simulink model "mp"  (R2017b)
settings: Solver=FixedStepAuto  StartTime=0.0  StopTime=0  FixedStep=stepSize  RelTol=1e-3
InitFcn:
  | mp_init
values from neighbouring files (symbols this model uses):
  carrierFreq = 5e6    (= 5000000)    [mp_init.m]
  dataRate = 1e6    (= 1000000)    [mp_init.m]
  detection_threshold = 150 + 2^11    (= 2198)    [mp_init.m]
  memSize = 1024    [mp_init.m]
  pilot_size = 2    [mp_init.m]
  sampleRate = clockRate    (= 40000000)    [mp_init.m]
  stepSize = 1/sampleRate    (= 2.5e-08)    [mp_init.m]
  wordLength = 12    [mp_init.m]
undefined symbols (not defined in the file or in its folder): AdvDSPBChannelOutDisplay, AdvDSPBDMemDisplay, dpoly, dspba_ChannelInVis, dspba_ChannelOutVis, dspba_internal_get_channel_ports, evalAionMaskParam, latency, UseDontCare, value
libraries: DSPBAPrim x75, DSPBABase x13, DSPBAControl x10, DSPBAFilters x3
(part 2 of 2)

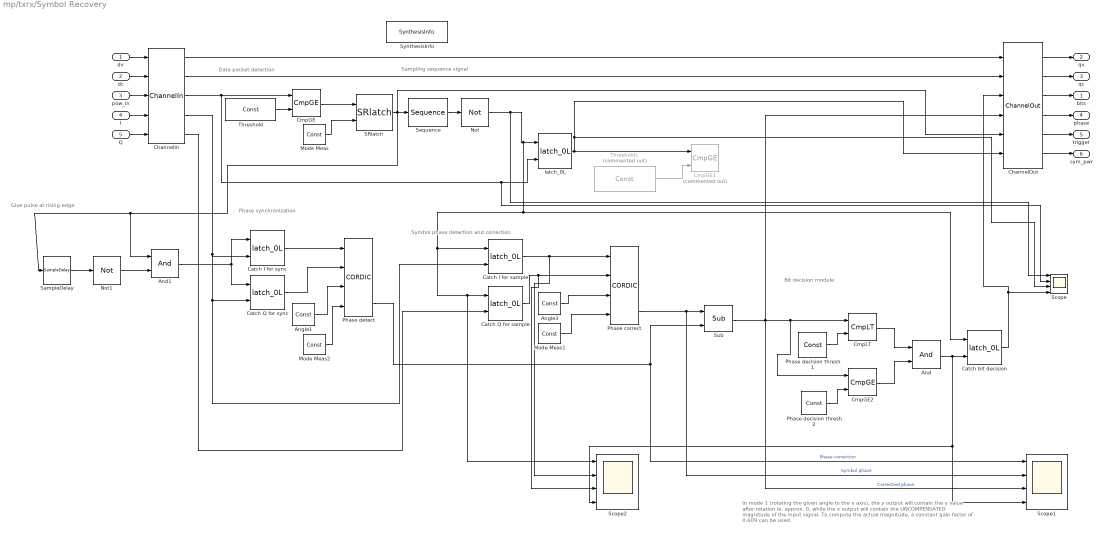
== system mp/txrx/Symbol Recovery ==
  note: Give pulse at rising edge
  note: Bit decision module
  note: Sampling sequence signal
  note: Data packet detection
  note: Symbol phase detection and correction
  note: Phase synchronization
  note: In mode 1 (rotating the given angle to the x axis),
      | the y output will contain the y value after rotation ie. approx. 0,
      | while the x output will contain the UNCOMPENSATED magnitude of the input signal.
      |
      | To compute the actual magnitude, a constant gain factor of 0.609 can be used.
  dv : Inport
  dc : Inport  Port=2
  pow_in : Inport  Port=3
  I : Inport  Port=4
  Q : Inport  Port=5
  And : DSPBAPrim/And  primtype=and  nInputs=2  nOutputs=1  omode=Inherit via internal rule  otype=sfix(16)  scale=2^-15  rndmethod=Unbiased  factor=1  satmethod=Symmetric  shift_vec=[0 1 2 -1]  value=0  inPortNames=[' '; ' '; ' '; ' '; ' '; ' '; ' '; ' '; ' '; ' '; ' '; ' '; ' '; ' '; ' '; ' '; ]  outPortNames=[' ']  dspbaimage=dspba_prim.jpg  text=fprintf('&');  style=Optimised  visibilities=8+2  version=20090407
  And1 : DSPBAPrim/And  primtype=and  nInputs=2  nOutputs=1  omode=Inherit via internal rule  otype=sfix(16)  scale=2^-15  rndmethod=Unbiased  factor=1  satmethod=Symmetric  shift_vec=[0 1 2 -1]  value=0  inPortNames=[' '; ' '; ' '; ' '; ' '; ' '; ' '; ' '; ' '; ' '; ' '; ' '; ' '; ' '; ' '; ' '; ]  outPortNames=[' ']  dspbaimage=dspba_prim.jpg  text=fprintf('&');  style=Optimised  visibilities=8+2  version=20090407
  Angle1 : DSPBAPrim/Const  primtype=const  nInputs=0  nOutputs=1  omode=Specify via dialog  otype=fixdt(1,28,14)  scale=1  rndmethod=Unbiased  factor=1  satmethod=Symmetric  shift_vec=[0 1 2 -1]  value=0  inPortNames=['+'; '+';]  outPortNames=[' ']  dspbaimage=dspba_prim.jpg  text=fprintf('%s', num2str(value));  style=Optimised  visibilities=8 + 1024  floatPrecision=float32_m23  version=20120820
  Angle3 : DSPBAPrim/Const  primtype=const  nInputs=0  nOutputs=1  omode=Specify via dialog  otype=fixdt(1,28,14)  scale=1  rndmethod=Unbiased  factor=1  satmethod=Symmetric  shift_vec=[0 1 2 -1]  value=0  inPortNames=['+'; '+';]  outPortNames=[' ']  dspbaimage=dspba_prim.jpg  text=fprintf('%s', num2str(value));  style=Optimised  visibilities=8 + 1024  floatPrecision=float32_m23  version=20120820
  Catch I for sample : DSPBAControl/latch_0L
  Catch I for sync : DSPBAControl/latch_0L
  Catch Q for sample : DSPBAControl/latch_0L
  Catch Q for sync : DSPBAControl/latch_0L
  Catch bit decision : DSPBAControl/latch_0L
  ChannelIn : DSPBAPrim/ChannelIn  primtype=channelin  nInputs=dspba_internal_get_channel_ports(gcb)  nOutputs=dspba_internal_get_channel_ports(gcb)  omode=Inherit via internal rule  otype=sfix(16)  scale=2^-15  rndmethod=Unbiased  factor=1  satmethod=Symmetric  shift_vec=[0 1 2 -1]  value=3  inPortNames=['v'; 'c'; '0'; '1'; '2'; '3'; '4'; '5'; '6'; '7'; '8'; '9'; 'A'; 'B'; 'D'; 'E'; 'F'; 'G'; 'H'; 'I'; 'J'; 'K'; 'L'; 'M'; 'N'; 'O'; 'P'; 'Q'; 'R'; 'S'; 'T'; 'U'; 'W'; 'X'; 'Y'; 'Z']  outPortNames=['v'; 'c'; '0'; '1'; '2'; '3'; '4'; '5'; '6'; '7'; '8'; '9'; 'A'; 'B'; 'D'; 'E'; 'F'; 'G'; 'H'; 'I'; 'J'; 'K'; 'L'; 'M'; 'N'; 'O'; 'P'; 'Q'; 'R'; 'S'; 'T'; 'U'; 'W'; 'X'; 'Y'; 'Z']  dspbaimage=dspba_prim.jpg  text=fprintf('In');  style=Optimised  dataSignals=3  foldingEnabled=off  channels=1  sampleRate=200  packetBeginPresent=off  packetBeginEnabled=off  visibilities=dspba_ChannelInVis(gcb)  latencyCorrection=0  scheduleOrigin=on  version=20141013
  ChannelOut : DSPBAPrim/ChannelOut  primtype=channelout  nInputs=dspba_internal_get_channel_ports(gcb)  nOutputs=dspba_internal_get_channel_ports(gcb)  omode=Inherit via internal rule  otype=sfix(16)  scale=2^-15  rndmethod=Unbiased  factor=1  satmethod=Symmetric  shift_vec=[0 1 2 -1]  value=4  inPortNames=['v'; 'c'; '0'; '1'; '2'; '3'; '4'; '5'; '6'; '7'; '8'; '9'; 'A'; 'B'; 'D'; 'E'; 'F'; 'G'; 'H'; 'I'; 'J'; 'K'; 'L'; 'M'; 'N'; 'O'; 'P'; 'Q'; 'R'; 'S'; 'T'; 'U'; 'W'; 'X'; 'Y'; 'Z']  outPortNames=['v'; 'c'; '0'; '1'; '2'; '3'; '4'; '5'; '6'; '7'; '8'; '9'; 'A'; 'B'; 'D'; 'E'; 'F'; 'G'; 'H'; 'I'; 'J'; 'K'; 'L'; 'M'; 'N'; 'O'; 'P'; 'Q'; 'R'; 'S'; 'T'; 'U'; 'W'; 'X'; 'Y'; 'Z']  dspbaimage=dspba_prim.jpg  text=fprintf('Out%s', AdvDSPBChannelOutDisplay(latency));  style=Optimised  dataSignals=4  foldingEnabled=off  channels=1  sampleRate=200  packetBeginPresent=off  packetBeginEnabled=off  visibilities=dspba_ChannelOutVis(gcb)  latency=3  latencyCorrection=0  version=20141013
  CmpGE : DSPBAPrim/CmpGE  primtype=cmpgte  nInputs=2  nOutputs=1  omode=boolean  otype=sfix(16)  scale=2^-15  rndmethod=Unbiased  factor=1  satmethod=Symmetric  shift_vec=[0 1 2 -1]  value=0  inPortNames=['a'; 'b';]  outPortNames=[' ']  dspbaimage=dspba_prim.jpg  text=fprintf('a>=b');  style=Optimised  visibilities=0  advOptions=[]  version=20130117
  CmpGE1 : DSPBAPrim/CmpGE  Commented=on  primtype=cmpgte  nInputs=2  nOutputs=1  omode=boolean  otype=sfix(16)  scale=2^-15  rndmethod=Unbiased  factor=1  satmethod=Symmetric  shift_vec=[0 1 2 -1]  value=0  inPortNames=['a'; 'b';]  outPortNames=[' ']  dspbaimage=dspba_prim.jpg  text=fprintf('a>=b');  style=Optimised  visibilities=0  advOptions=[]  version=20130117
  CmpGE2 : DSPBAPrim/CmpGE  primtype=cmpgte  nInputs=2  nOutputs=1  omode=boolean  otype=sfix(16)  scale=2^-15  rndmethod=Unbiased  factor=1  satmethod=Symmetric  shift_vec=[0 1 2 -1]  value=0  inPortNames=['a'; 'b';]  outPortNames=[' ']  dspbaimage=dspba_prim.jpg  text=fprintf('a>=b');  style=Optimised  visibilities=0  advOptions=[]  version=20130117
  CmpLT : DSPBAPrim/CmpLT  primtype=cmplt  nInputs=2  nOutputs=1  omode=boolean  otype=sfix(16)  scale=2^-15  rndmethod=Unbiased  factor=1  satmethod=Symmetric  shift_vec=[0 1 2 -1]  value=0  inPortNames=['a'; 'b';]  outPortNames=[' ']  dspbaimage=dspba_prim.jpg  text=fprintf('a<b');  style=Optimised  visibilities=0  advOptions=[]  version=20130117
  Mode Meas : DSPBAPrim/Const  primtype=const  nInputs=0  nOutputs=1  omode=boolean  otype=ufix(1)  scale=1  rndmethod=Unbiased  factor=1  satmethod=Symmetric  shift_vec=[0 1 2 -1]  value=0  inPortNames=['+'; '+';]  outPortNames=[' ']  dspbaimage=dspba_prim.jpg  text=fprintf('%s', num2str(value));  style=Optimised  visibilities=8 + 1024  floatPrecision=float32_m23  version=20120820
  Mode Meas1 : DSPBAPrim/Const  primtype=const  nInputs=0  nOutputs=1  omode=boolean  otype=ufix(1)  scale=1  rndmethod=Unbiased  factor=1  satmethod=Symmetric  shift_vec=[0 1 2 -1]  value=1  inPortNames=['+'; '+';]  outPortNames=[' ']  dspbaimage=dspba_prim.jpg  text=fprintf('%s', num2str(value));  style=Optimised  visibilities=8 + 1024  floatPrecision=float32_m23  version=20120820
  Mode Meas2 : DSPBAPrim/Const  primtype=const  nInputs=0  nOutputs=1  omode=boolean  otype=ufix(1)  scale=1  rndmethod=Unbiased  factor=1  satmethod=Symmetric  shift_vec=[0 1 2 -1]  value=1  inPortNames=['+'; '+';]  outPortNames=[' ']  dspbaimage=dspba_prim.jpg  text=fprintf('%s', num2str(value));  style=Optimised  visibilities=8 + 1024  floatPrecision=float32_m23  version=20120820
  Not : DSPBAPrim/Not  primtype=not  nInputs=1  nOutputs=1  omode=Inherit via internal rule  otype=sfix(16)  scale=2^-15  rndmethod=Unbiased  factor=1  satmethod=Symmetric  shift_vec=[0 1 2 -1]  value=0  inPortNames=[' '; ' ';]  outPortNames=[' ']  dspbaimage=dspba_prim.jpg  text=fprintf('~');  style=Optimised  visibilities=8  version=20090407
  Not1 : DSPBAPrim/Not  primtype=not  nInputs=1  nOutputs=1  omode=Inherit via internal rule  otype=sfix(16)  scale=2^-15  rndmethod=Unbiased  factor=1  satmethod=Symmetric  shift_vec=[0 1 2 -1]  value=0  inPortNames=[' '; ' ';]  outPortNames=[' ']  dspbaimage=dspba_prim.jpg  text=fprintf('~');  style=Optimised  visibilities=8  version=20090407
  Phase correct : DSPBAPrim/CORDIC  primtype=cordic  nInputs=4  nOutputs=3  omode=Specify via dialog  otype=fixdt(1,28,14)  scale=1  rndmethod=Unbiased  factor=1  satmethod=Symmetric  shift_vec=[0 1 2 -1]  value=0  inPortNames=['x'; 'y'; 'p'; 'v']  outPortNames=['x'; 'y'; 'p']  dspbaimage=dspba_prim.jpg  text=fprintf('cordic');  style=Optimised  visibilities=8  version=20090407
  Phase decision thresh 1 : DSPBAPrim/Const  primtype=const  nInputs=0  nOutputs=1  omode=Specify via dialog  otype=fixdt(1,wordLength,10)  scale=1  rndmethod=Unbiased  factor=1  satmethod=Symmetric  shift_vec=[0 1 2 -1]  value=pi/2  inPortNames=['+'; '+';]  outPortNames=[' ']  dspbaimage=dspba_prim.jpg  text=fprintf('%s', num2str(value));  style=Optimised  visibilities=8 + 1024  floatPrecision=float32_m23  version=20120820
  Phase decision thresh 2 : DSPBAPrim/Const  primtype=const  nInputs=0  nOutputs=1  omode=Specify via dialog  otype=fixdt(1,wordLength,10)  scale=1  rndmethod=Unbiased  factor=1  satmethod=Symmetric  shift_vec=[0 1 2 -1]  value=-pi/2  inPortNames=['+'; '+';]  outPortNames=[' ']  dspbaimage=dspba_prim.jpg  text=fprintf('%s', num2str(value));  style=Optimised  visibilities=8 + 1024  floatPrecision=float32_m23  version=20120820
  Phase detect : DSPBAPrim/CORDIC  primtype=cordic  nInputs=4  nOutputs=3  omode=Specify via dialog  otype=fixdt(1,28,14)  scale=1  rndmethod=Unbiased  factor=1  satmethod=Symmetric  shift_vec=[0 1 2 -1]  value=0  inPortNames=['x'; 'y'; 'p'; 'v']  outPortNames=['x'; 'y'; 'p']  dspbaimage=dspba_prim.jpg  text=fprintf('cordic');  style=Optimised  visibilities=8  version=20090407
  SRlatch : DSPBAControl/SRlatch
  SampleDelay : DSPBAPrim/SampleDelay  primtype=sampdelay  nInputs=1  nOutputs=1  omode=Inherit via internal rule  otype=sfix(16)  scale=2^-15  rndmethod=Unbiased  factor=1  satmethod=Symmetric  shift_vec=[0 1 2 -1]  value=1  inPortNames=[' '; ' ';]  outPortNames=[' ']  dspbaimage=dspba_prim.jpg  text=dpoly(1, eye(1,value+1), 'z')  style=Optimised  visibilities=8 + 1024 + 2^17 + 2^18  flexible=off  slackgroup=0  augmented=0  version=20090407  advOptions=[]
  Scope : Scope  NumInputPorts=4
  Scope1 : Scope  NumInputPorts=4
  Scope2 : Scope  NumInputPorts=4
  Sequence : DSPBAPrim/Sequence  primtype=sequencer  nInputs=1  nOutputs=1  omode=Inherit via internal rule  otype=ufix(16)  scale=2^-0  rndmethod=Unbiased  factor=1  satmethod=Symmetric  shift_vec=[0 1 2 -1]  value=[39-4 1 40]  inPortNames=[' '; ' ';]  outPortNames=[' ']  dspbaimage=dspba_prim.jpg  text=fprintf('seq\n[%d %d %d]', value(1), value(2), value(3));  style=Optimised  visibilities=1024  version=20090407
  Sub : DSPBAPrim/Sub  primtype=sub  nInputs=2  nOutputs=1  omode=Inherit via internal rule with word growth  otype=sfix(16)  scale=2^-15  rndmethod=Unbiased  factor=1  satmethod=Symmetric  shift_vec=[0 1 2 -1]  value=0  inPortNames=['+'; '-';]  outPortNames=[' ']  dspbaimage=dspba_prim.jpg  text=fprintf('-');  style=Optimised  visibilities=8+2^17+2^18  floatRounding=correct  advOptions=[]  version=20130115
  SynthesisInfo : DSPBAPrim/SynthesisInfo  primtype=synthinfo  nInputs=0  nOutputs=0  omode=Inherit via internal rule  otype=sfix(16)  scale=2^-15  rndmethod=Truncate  factor=1  satmethod=Symmetric  shift_vec=[0 1 2 -1]  value=99  inPortNames=[' '; ' ';]  outPortNames=[' ']  dspbaimage=dspba_prim_ctrl.jpg  text=fprintf('Style=%s', style);  style=Scheduled  visibilities=2^17+2^18+2^19+2^20  constraintInUse=off  constraintRelation=>  constraintLimit=2  bitAccurate=off  version=20150220
  Threshold : DSPBAPrim/Const  primtype=const  nInputs=0  nOutputs=1  omode=Specify via dialog  otype=fixdt(1,65,22)  scale=1  rndmethod=Unbiased  factor=1  satmethod=Symmetric  shift_vec=[0 1 2 -1]  value=detection_threshold  inPortNames=['+'; '+';]  outPortNames=[' ']  dspbaimage=dspba_prim.jpg  text=fprintf('%s', num2str(value));  style=Optimised  visibilities=8 + 1024  floatPrecision=float32_m23  version=20120820
  Threshold1 : DSPBAPrim/Const  Commented=on  primtype=const  nInputs=0  nOutputs=1  omode=Specify via dialog  otype=fixdt(1,wordLength)  scale=1  rndmethod=Unbiased  factor=1  satmethod=Symmetric  shift_vec=[0 1 2 -1]  value=detection_threshold/2  inPortNames=['+'; '+';]  outPortNames=[' ']  dspbaimage=dspba_prim.jpg  text=fprintf('%s', num2str(value));  style=Optimised  visibilities=8 + 1024  floatPrecision=float32_m23  version=20120820
  latch_0L : DSPBAControl/latch_0L
  bits : Outport
  qv : Outport  Port=2
  qc : Outport  Port=3
  phase : Outport  Port=4
  trigger : Outport  Port=5
  sym_pwr : Outport  Port=6
  wires:
  ChannelOut/3 -> bits/1
  dv/1 -> ChannelIn/1
  ChannelOut/1 -> qv/1
  dc/1 -> ChannelIn/2
  ChannelOut/2 -> qc/1
  pow_in/1 -> ChannelIn/3
  ChannelIn/3 -> CmpGE/1, Scope/2, latch_0L/2
  Threshold/1 -> CmpGE/2
  ChannelIn/1 -> ChannelOut/1
  ChannelIn/2 -> ChannelOut/2
  CmpGE/1 -> SRlatch/1
  Mode Meas/1 -> SRlatch/2
  SRlatch/1 -> And1/1, SampleDelay/1, ChannelOut/5, Sequence/1
  Sequence/1 -> Not/1
  Not/1 -> latch_0L/1, Catch bit decision/1, Scope2/1, Catch Q for sample/1, Catch I for sample/1, Scope/1
  latch_0L/1 -> ChannelOut/6, Scope/3, CmpGE1/1
  I/1 -> ChannelIn/4
  Q/1 -> ChannelIn/5
  Mode Meas1/1 -> Phase correct/4
  ChannelIn/4 -> Catch I for sync/2, Catch I for sample/2, Catch Q for sync/2
  ChannelIn/5 -> Catch Q for sample/2
  Catch I for sample/1 -> Scope2/2, Phase correct/1
  Catch Q for sample/1 -> Scope2/3, Phase correct/2
  ChannelOut/4 -> phase/1
  Threshold1/1 -> CmpGE1/2
  ChannelOut/5 -> trigger/1
  ChannelOut/6 -> sym_pwr/1
  Mode Meas2/1 -> Phase detect/4
  Catch I for sync/1 -> Phase detect/1
  Catch Q for sync/1 -> Phase detect/2
  Angle1/1 -> Phase detect/3
  Phase detect/3 -> Scope1/1, Sub/2  "Phase correction"
  Phase decision thresh 1/1 -> CmpLT/2
  Phase decision thresh 2/1 -> CmpGE2/2
  CmpLT/1 -> And/1
  CmpGE2/1 -> And/2
  And/1 -> Scope2/4, Scope1/4, Catch bit decision/2
  Catch bit decision/1 -> ChannelOut/3, Scope/4
  Angle3/1 -> Phase correct/3
  Phase correct/3 -> Scope1/2, Sub/1  "Symbol phase"
  Sub/1 -> ChannelOut/4, Scope1/3, CmpGE2/1, CmpLT/1  "Correctied phase"
  SampleDelay/1 -> Not1/1
  Not1/1 -> And1/2
  And1/1 -> Catch I for sync/1, Catch Q for sync/1
